simulink model "ALBERT02"  (R2024b)
settings: Solver=VariableStepAuto  StartTime=0.0  StopTime=16  RelTol=1e-3
undefined symbols (not defined in the file or in its folder): K1
settings Model: Creator=felixzauner  LastModifiedBy=felixzauner

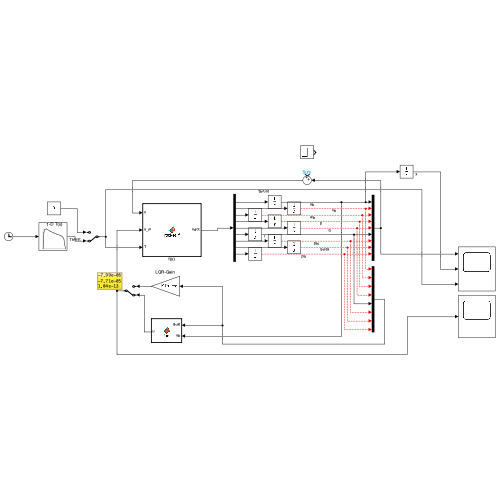
[thumbnail: Simulink's stored preview of the top-level diagram]
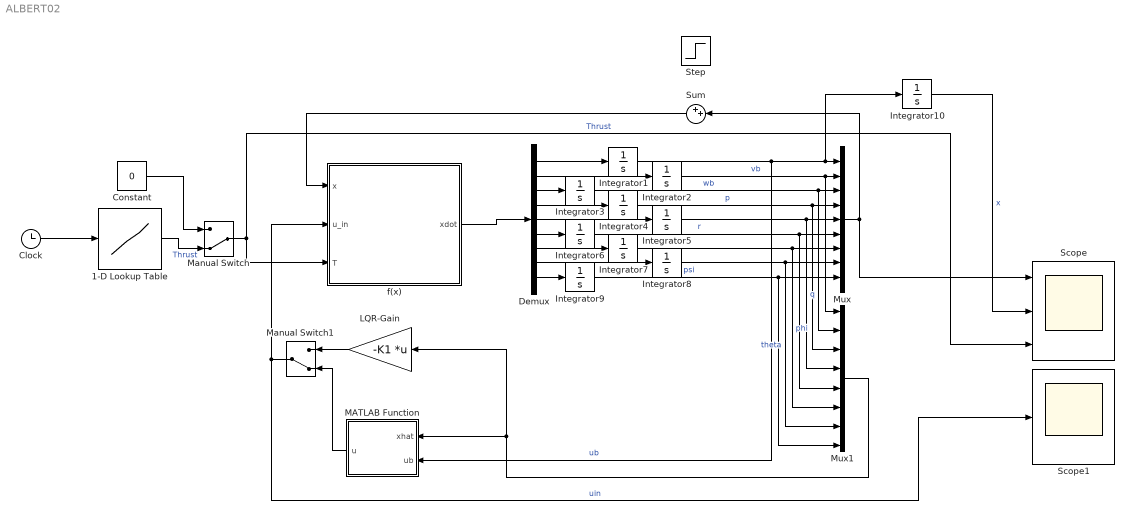
== system ALBERT02 ==
  1-D Lookup Table : Lookup_n-D  NumberOfTableDimensions=1  BreakpointsForDimension1=[0 0.02 0.05 0.10 0.20 0.40 0.60 0.80 1.00 1.10 1.20 1.25 1.30]  Table=[0 60 140 165 170 150 135 125 115 105 90 40 0]  ExtrapMethod=Clip  InternalRulePriority=Speed  RndMeth=Simplest
  Clock : Clock
  Constant : Constant  Value=0
  Demux : Demux  Outputs=9
  Integrator{1..10} (10 alike) : Integrator
  LQR-Gain : Gain  Gain=-K1  Multiplication=Matrix(K*u) (u vector)
  MATLAB Function : MATLAB Function  TreatAsAtomicUnit=on
  Manual Switch : ManualSwitch  CurrentSetting=0
  Manual Switch1 : ManualSwitch  CurrentSetting=0
  Mux : Mux  Inputs=9
  Mux1 : Mux  Inputs=8
  Scope : Scope  NumInputPorts=3
  Scope1 : Scope
  Step : Step  Time=2  After=0.1  SampleTime=0
  Sum : Sum  Inputs=++|
  f(x) : MATLAB Function  TreatAsAtomicUnit=on
  wires:
  Clock/1 -> 1-D Lookup Table/1
  1-D Lookup Table/1 -> Manual Switch/2  "Thrust"
  Constant/1 -> Manual Switch/1
  LQR-Gain/1 -> Manual Switch1/1
  Manual Switch1/1 -> f(x)/2(u_in), Scope1/1  "uin"
  Integrator5/1 -> Mux1/4, Mux/5  "q"
  Integrator4/1 -> Mux1/3, Mux/4  "p"
  Integrator1/1 -> Integrator10/1, Mux/1, MATLAB Function/2(ub)  "ub"
  Demux/5 -> Integrator5/1
  Integrator8/1 -> Mux1/7, Mux/8  "theta"
  Integrator3/1 -> Mux1/2, Mux/3  "wb"
  f(x)/1(xdot) -> Demux/1
  Demux/7 -> Integrator7/1
  Demux/3 -> Integrator3/1
  Demux/4 -> Integrator4/1
  Integrator7/1 -> Mux1/6, Mux/7  "phi"
  Integrator2/1 -> Mux1/1, Mux/2  "vb"
  Demux/1 -> Integrator1/1
  Demux/2 -> Integrator2/1
  Demux/8 -> Integrator8/1
  Demux/6 -> Integrator6/1
  Manual Switch/1 -> Scope/3, f(x)/3(T)  "Thrust"
  MATLAB Function/1(u) -> Manual Switch1/2
  Demux/9 -> Integrator9/1
  Integrator9/1 -> Mux1/8, Mux/9  "psi"
  Mux1/1 -> MATLAB Function/1(xhat), LQR-Gain/1
  Mux/1 -> Scope/1, Sum/2
  Sum/1 -> f(x)/1(x)
  Integrator10/1 -> Scope/2  "x"
  Integrator6/1 -> Mux1/5, Mux/6  "r"

== matlab function ALBERT02/MATLAB Function ==
  data: xhat input; u output; ub input; K_array parameter
function u = fcn(xhat, ub, K_array)

m = 3;
n= 8;

u_values = 10:10:200;
K_fun = cell(m,n);

for i = 1:m
    for j = 1:n
        kij_values = squeeze(K_array(i,j,:));
        K_fun{i,j} = griddedInterpolant(u_values, kij_values, 'linear');
    end
end

K_eval = zeros(3,8);

for i = 1:m
    for j = 1:n
        %K_eval(i,j) = polyval(P{i,j}, ub_val);
        K_eval(i,j) = K_fun{i,j}(ub);
    end
end
u = -K_eval * xhat;
end

== matlab function ALBERT02/f(x) ==
  data: x input; xdot output; u_in input; T input
% Nonlinear Function for a Rocket
function xdot = rocket_f(x, u_in,T)
% x = [u v w p q r phi theta psi]'
% u_in = [delta_eta delta_zeta delta_r T]' 

% Define Parameters
% --- Geometry / environment ---
g0   = 9.81;        % m/s^2
rho0 = 1.225;       % kg/m^3 (sea level)
S    = 0.010;       % m^2  reference area
d    = 0.10;        % m    reference diameter

% --- Mass / inertia ---
m  = 1.6;          % kg
Ix = 0.005;         % kg*m^2
Iy = 0.020;         % kg*m^2 
Iz = 0.020;         % kg*m^2

% --- Aerodynamic force coeffs ---
CA0       = 0.093292905;   % axial (drag-like)
CA_kalpha = 0.0593605;   % axial vs alpha
CA_kbeta  = 0.0593605;   % axial vs beta

% --- Moment coeffs ---
Cl_delta = 0.229;    % roll control effectiveness
Clp      = -10;     % roll damping
Cm_alpha = 2.6130694;    % pitch stability derivative
Cm_delta = 2.7716625;    % pitch control effectiveness
Cmq      = -24.89;     % pitch damping
Cn_beta  = 2.6130694;     % yaw stability derivative
Cn_delta = 2.7716625;     % yaw control effectiveness
Cnr      = -24.89;     % yaw damping

CY_beta = -2.0577392;
CY_zeta = -0.6508215;

CZ_alpha = -2.0577392;
CZ_eta = -0.6508215;

% --- Reference points ---
xcm  = 0.60;        % m 
xref = 0.5;        % m 

% --- unpack state ---
ub    = x(1);  vb = x(2);  wb = x(3);       
p     = x(4);  q  = x(5);  r  = x(6);
phi   = x(7);  theta = x(8); psi = x(9);

% --- unpack inputs ---
delta_eta  = u_in(1);
delta_zeta = u_in(2);
delta_r    = u_in(3);


% --- derived quantities ---
V = sqrt(ub^2 + vb^2 + wb^2+ 1e-9^2);  % avoid div0
alpha = atan2(wb,ub);
beta  = asin(vb / V); 
alpha_total = atan2(sqrt(vb^2 + wb^2), ub);
% Dynamic pressure q = 1/2 p V^2 for moments
Qdyn = 0.5*rho0*V^2;


CA = CA0 + CA_kalpha*alpha + CA_kbeta*beta;
CN = CY_beta*beta + CY_zeta*delta_zeta + CZ_alpha*alpha + CZ_eta*delta_eta;
% Build direct force coefficiants
CNy = CN * -vb / sqrt(vb^2 + wb^2 + 1e-9);
CNz = CN * -wb / sqrt(vb^2 + wb^2 + 1e-9);

% Aerodynamic forces 
FAxb = -Qdyn * CA  * S;
FAyb =  Qdyn * CNy * S;
FAzb =  Qdyn * CNz * S;

% --- thrust in body ---
FPxb = T;  FPyb = 0;  FPzb = 0;

% --- gravity in body: Fg_b = R_nb' * [0;0;mg] in NED ---
% NED: gravity in nav frame is [0;0; +m*g] (Down positive)
Fg_n = [-m*g0; 0;0];

% Rotation matrix R_b^n (ZYX) and R_n^b = (R_b^n)'
cphi = cos(phi); sphi = sin(phi);
cth  = cos(theta); sth = sin(theta);
cps  = cos(psi); sps  = sin(psi);

% ZYX: body->nav (matches common aerospace convention)
R_b_n = [ cth*cps,  sphi*sth*cps - cphi*sps,  cphi*sth*cps + sphi*sps;
          cth*sps,  sphi*sth*sps + cphi*cps,  cphi*sth*sps - sphi*cps;
          -sth,     sphi*cth,              cphi*cth ];
R_n_b = R_b_n';

Fg_b = R_n_b * Fg_n;
Fgxb = Fg_b(1); Fgyb = Fg_b(2); Fgzb = Fg_b(3);

% --- total forces ---
Fx = FAxb + FPxb + Fgxb;
Fy = FAyb + FPyb + Fgyb;
Fz = FAzb + FPzb + Fgzb;

% --- moment coefficients  ---
Cl = Cl_delta*delta_r + (d/(2*V))*Clp*p;

% Pitch & yaw moment coefficients
Cmref = Cm_alpha*alpha + Cm_delta*delta_eta;
Cnref = Cn_beta *beta  + Cn_delta*delta_zeta;

Cm = Cmref - CNz*((xcm-xref)/d) + (d/(2*V))*(Cmq + Cm_alpha)*q;
Cn = Cnref - CNy*((xcm-xref)/d) + (d/(2*V))*(Cnr + Cn_beta )*r;

LA = Qdyn * Cl * S * d;
MA = Qdyn * Cm * S * d;
NA = Qdyn * Cn * S * d;

% Propulsion moments 
Lp = 0; Mp = 0; Np = 0;

% --- translational dynamics in body ---
udot = Fx/m - (q*wb - r*vb);
vdot = Fy/m - (r*ub - p*wb);
wdot = Fz/m - (p*vb - q*ub);

% --- rotational dynamics ---
pdot = (LA + Lp - q*r*(Iz - Iy))/Ix;
qdot = (MA + Mp - r*p*(Ix - Iz))/Iy;
rdot = (NA + Np - p*q*(Iy - Ix))/Iz;

% --- Euler kinematics ---
phidot   = p + (q*sin(phi) + r*cos(phi))*tan(theta);
thetadot = q*cos(phi) - r*sin(phi);
psidot   = (q*sin(phi) + r*cos(phi))/cos(theta);

xdot = [udot vdot wdot pdot qdot rdot phidot thetadot psidot];
end
